simulink subsystem "quantile_lut_controller"  (R2024b)
settings: Solver=VariableStepAuto  StartTime=0.0  StopTime=10.0  RelTol=1e-3
undefined symbols (not defined in the file or in its folder): baro_lut, const_brake, controller_rate, observer_rate
settings Model: Creator=yevge  LastModifiedBy=yevge

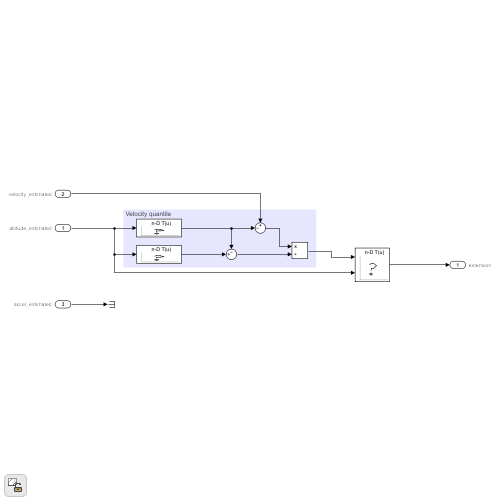
[thumbnail: Simulink's stored preview of the top-level diagram]
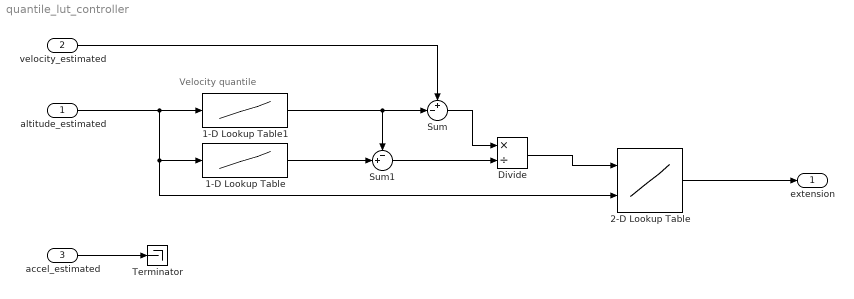
== system quantile_lut_controller ==
  note: Velocity quantile
  altitude_estimated : Inport  Unit=m  PortDimensions=1  SampleTime=1/observer_rate
  velocity_estimated : Inport  Port=2  Unit=m/s  PortDimensions=1  SampleTime=1/observer_rate
  accel_estimated : Inport  Port=3  Unit=m/s^2  PortDimensions=1  SampleTime=1/observer_rate
  1-D Lookup Table : Lookup_n-D  NumberOfTableDimensions=1  DataSpecification=Lookup table object  LookupTableObject=upper_bound_lut  BreakpointsForDimension1=[-5:5]  Table=tanh([-5:5])  InternalRulePriority=Speed  RndMeth=Simplest
  1-D Lookup Table1 : Lookup_n-D  NumberOfTableDimensions=1  DataSpecification=Lookup table object  LookupTableObject=lower_bound_lut  BreakpointsForDimension1=[-5:5]  Table=tanh([-5:5])  InternalRulePriority=Speed  RndMeth=Simplest
  2-D Lookup Table : Lookup_n-D  DataSpecification=Lookup table object  LookupTableObject=quantile_lut  BreakpointsForDimension1=baro_lut.vel  BreakpointsForDimension2=baro_lut.alt  Table=baro_lut{:, :}  InternalRulePriority=Speed  RndMeth=Simplest
      settings: InputPortMap=u0,u1
  Divide : Product  Inputs=*/
  Sum : Sum  Inputs=+-|
  Sum1 : Sum  Inputs=-+|
  Terminator : Terminator
  extension : Outport  Unit=1  PortDimensions=1  SampleTime=1/controller_rate  InitialOutput=const_brake
  wires:
  accel_estimated/1 -> Terminator/1
  2-D Lookup Table/1 -> extension/1
  altitude_estimated/1 -> 2-D Lookup Table/2, 1-D Lookup Table/1, 1-D Lookup Table1/1
  1-D Lookup Table1/1 -> Sum1/1, Sum/2
  1-D Lookup Table/1 -> Sum1/2
  Sum/1 -> Divide/1
  Sum1/1 -> Divide/2
  velocity_estimated/1 -> Sum/1
  Divide/1 -> 2-D Lookup Table/1
